simulink library "LIB_DYN"  (Simulink 8.8)
settings: Solver=ode45  StartTime=0.0  StopTime=10.0  RelTol=1e-3  EnableMultiTasking=on
libraries: LIB_ROT x5
settings Model: Creator=alger  LastModifiedBy=alger

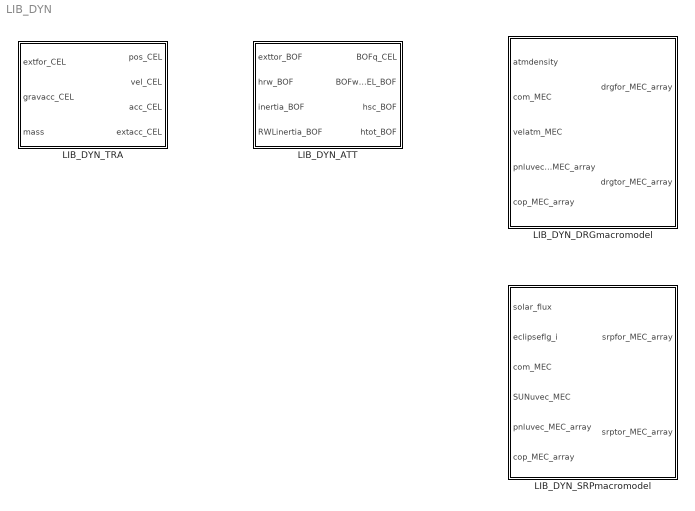
== system LIB_DYN ==
  LIB_DYN_ATT : Subsystem  mask(Integrates Attitude States){BOFq_CEL_ini=0, h_BOF_ini=0, zero_tol=0}
      mask prompts: BOFq_CEL_ini "inital Body to Cel Frame Quaternion"; h_BOF_ini "inital angular momentum of body frame"; zero_tol "near zero tolerance"
      mask help:
      | Integrates attitude states of a spacecraft (or part of a spacecraft) in the Body Frame w.r.t an inertial celestial frame
      |
      | Inputs
      | exttor_BOF: exteral torques acting on the spacecraft [N]
      | hrw_BOF: momentum exchange with other components of the spacecraft e.g. reaction wheels [Nms]
      | inertia_BOF: current inertia of the spacecraft in body frame[kg/m^2]
      | RWinertia_BOF: current inertia of other components of the spacecraft e.g. reaction wheels[kg/m^2]
      |
      | Outputs
      | BOFq_CEL: quaterion relating celestial and body frames[-]
      | BOFw_rel_CEL_BOF: rates of rotation between celestial and body frames expressed in terms of the BOF frame [rad/s]
      | hsc_BOF: angular momentum of spaceccraft (e.g. no momentum from reaction wheels)[Nms]
      | htot_BOF:angular momentum of spacecraft and any exchanged momentum[Nms]
  "LIB_DYN_DRGmacromodel " : Subsystem  mask{N=6, pnlarea_array=[0.1, 0.1, 0.1, 0.1, 0.1, 0.1], pnlcd_array=[0.5, 0.5, 0.5, 0.5, 0.5, 0.5]}
      mask prompts: N "Number of panels"; pnlarea_array "Surface area for each panel"; pnlcd_array "Drag coeffiecent for each panel"
  LIB_DYN_SRPmacromodel : Subsystem  mask{N=6, C=0, pnlarea_array=[0.1, 0.1, 0.1, 0.1, 0.1, 0.1], pnlcrd_array=[0.15, 0.15, 0.15, 0.15, 0.15, 0.15], pnlcrs_array=[0.75, 0.75, 0.75, 0.75, 0.75, 0.75]}
      mask prompts: N "Number of panels"; C "Speed of light constant (m/s)"; pnlarea_array "Surface area for each panel"; pnlcrd_array "diffuse coefficentfor each panel"; pnlcrs_array "specular coefficent for each panel"
      mask help: absorbed coefficent is computed based on 1-(crd +crs)
  LIB_DYN_TRA : Subsystem  mask(Integrates translational states){pos_CEL_ini=0, vel_CEL_ini=0}
      mask prompts: pos_CEL_ini "Initial position in inertial celestial frame  [m]"; vel_CEL_ini "Intial velocity in an inertial celestial frame[m/s]"
      mask help:
      | integrates translational states in an inertial celestial frame using integrator blocks from matlab.
      |
      | Inputs
      | extfor_CEL: External forces acting on the spacecraft expressed in a inertial Celestial frame [N]
      | gravacc_CEL: Acceleration due to gravity of the planetary body the spacecraft is orbiting [m/s^2]
      | mass:  mass of the spacecraft
      |
      | Ouptuts
      | pos_CEL: integrated position of spacecraft in an inertial celestial frame [m]
      | vel_CEL: integrated velocity of spacecraft in an inertial celestial frame[m/s]
      | acc_CEL: net acceleration of spacecraft in an inertial celestial frame[m/^s]
      | extacc_CEL: accleration of spacecraft due to external forces only in an inertial celestial frame[m/s^2]

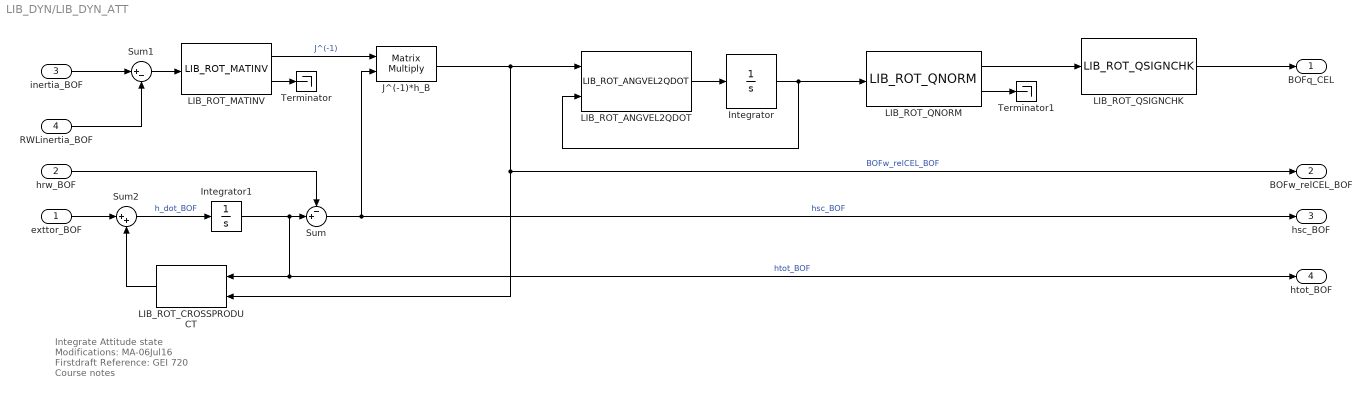
== system LIB_DYN/LIB_DYN_ATT ==
  note: Integrate Attitude state
      |
      | Modifications:
      | MA-06Jul16 Firstdraft
      |
      | Reference:
      | GEI 720 Course notes
  exttor_BOF : Inport  PortDimensions=3
  hrw_BOF : Inport  Port=2  PortDimensions=3
  inertia_BOF : Inport  Port=3  PortDimensions=[3,3]
  RWLinertia_BOF : Inport  Port=4  PortDimensions=[3,3]
  Integrator : Integrator  InitialCondition=BOFq_CEL_ini
  Integrator1 : Integrator  InitialCondition=h_BOF_ini
  J^(-1)*h_B : Product  Multiplication=Matrix(*)  RndMeth=Zero
  LIB_ROT_ANGVEL2QDOT : LIB_ROT/LIB_ROT_ANGVEL2QDOT
  LIB_ROT_CROSSPRODUCT : LIB_ROT/LIB_ROT_CROSSPRODUCT
  "LIB_ROT_MATINV " : LIB_ROT/LIB_ROT_MATINV   tol=zero_tol
  LIB_ROT_QNORM : LIB_ROT/LIB_ROT_QNORM  zero_tol=zero_tol
  LIB_ROT_QSIGNCHK : LIB_ROT/LIB_ROT_QSIGNCHK  tol=zero_tol
  Sum : Sum  Inputs=-+|
  Sum1 : Sum  Inputs=|+-
  Sum2 : Sum  Inputs=|++
  Terminator : Terminator
  Terminator1 : Terminator
  BOFq_CEL : Outport  PortDimensions=4
  BOFw_relCEL_BOF : Outport  Port=2  PortDimensions=3
  hsc_BOF : Outport  Port=3  PortDimensions=3
  htot_BOF : Outport  Port=4  PortDimensions=3
  wires:
  inertia_BOF/1 -> Sum1/1
  RWLinertia_BOF/1 -> Sum1/2
  "LIB_ROT_MATINV "/1 -> J^(-1)*h_B/1  "J^(-1)"
  Sum1/1 -> "LIB_ROT_MATINV "/1
  hrw_BOF/1 -> Sum/1
  exttor_BOF/1 -> Sum2/1
  Sum2/1 -> Integrator1/1  "h_dot_BOF"
  Integrator1/1 -> LIB_ROT_CROSSPRODUCT/1, htot_BOF/1, Sum/2  "htot_BOF"
  J^(-1)*h_B/1 -> BOFw_relCEL_BOF/1, LIB_ROT_CROSSPRODUCT/2, LIB_ROT_ANGVEL2QDOT/1  "BOFw_relCEL_BOF"
  Sum/1 -> J^(-1)*h_B/2, hsc_BOF/1  "hsc_BOF"
  LIB_ROT_CROSSPRODUCT/1 -> Sum2/2
  "LIB_ROT_MATINV "/2 -> Terminator/1
  LIB_ROT_ANGVEL2QDOT/1 -> Integrator/1
  Integrator/1 -> LIB_ROT_QNORM/1, LIB_ROT_ANGVEL2QDOT/2
  LIB_ROT_QNORM/1 -> LIB_ROT_QSIGNCHK/1
  LIB_ROT_QNORM/2 -> Terminator1/1
  LIB_ROT_QSIGNCHK/1 -> BOFq_CEL/1

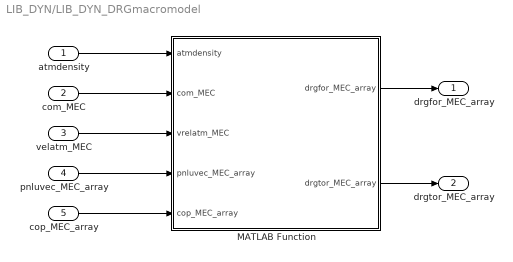
== system LIB_DYN/LIB_DYN_DRGmacromodel  ==
  atmdensity : Inport  Unit=kg/m^3  PortDimensions=1
  com_MEC : Inport  Port=2  Unit=m  PortDimensions=3
  velatm_MEC : Inport  Port=3  PortDimensions=3
  pnluvec_MEC_array : Inport  Port=4  PortDimensions=[3, N]  LockScale=on
  cop_MEC_array : Inport  Port=5  Unit=m  PortDimensions=[3, N]
  MATLAB Function : MATLAB Function  TreatAsAtomicUnit=on
  drgfor_MEC_array : Outport  PortDimensions=[3, N]
  drgtor_MEC_array : Outport  Port=2  PortDimensions=[3, N]
  wires:
  cop_MEC_array/1 -> MATLAB Function/5(cop_MEC_array)
  atmdensity/1 -> MATLAB Function/1(atmdensity)
  com_MEC/1 -> MATLAB Function/2(com_MEC)
  velatm_MEC/1 -> MATLAB Function/3(vrelatm_MEC)
  pnluvec_MEC_array/1 -> MATLAB Function/4(pnluvec_MEC_array)
  MATLAB Function/2(drgtor_MEC_array) -> drgtor_MEC_array/1
  MATLAB Function/1(drgfor_MEC_array) -> drgfor_MEC_array/1

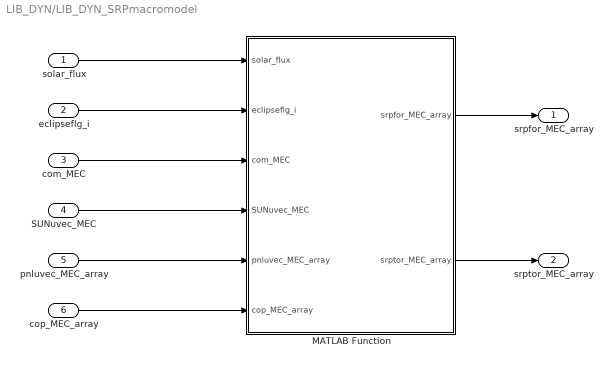
== system LIB_DYN/LIB_DYN_SRPmacromodel ==
  solar_flux : Inport  Unit=kg/m^3  PortDimensions=1
  eclipseflg_i : Inport  Port=2  Unit=kg/m^3  PortDimensions=1
  com_MEC : Inport  Port=3  Unit=m  PortDimensions=3
  SUNuvec_MEC : Inport  Port=4  PortDimensions=3
  pnluvec_MEC_array : Inport  Port=5  PortDimensions=[3, N]  LockScale=on
  cop_MEC_array : Inport  Port=6  Unit=m  PortDimensions=[3, N]
  MATLAB Function : MATLAB Function  TreatAsAtomicUnit=on
  srpfor_MEC_array : Outport  PortDimensions=[3, N]
  srptor_MEC_array : Outport  Port=2  PortDimensions=[3, N]
  wires:
  MATLAB Function/1(srpfor_MEC_array) -> srpfor_MEC_array/1
  MATLAB Function/2(srptor_MEC_array) -> srptor_MEC_array/1
  pnluvec_MEC_array/1 -> MATLAB Function/5(pnluvec_MEC_array)
  SUNuvec_MEC/1 -> MATLAB Function/4(SUNuvec_MEC)
  com_MEC/1 -> MATLAB Function/3(com_MEC)
  solar_flux/1 -> MATLAB Function/1(solar_flux)
  cop_MEC_array/1 -> MATLAB Function/6(cop_MEC_array)
  eclipseflg_i/1 -> MATLAB Function/2(eclipseflg_i)

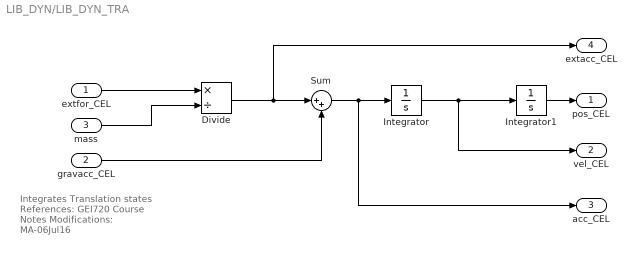
== system LIB_DYN/LIB_DYN_TRA ==
  note: Integrates Translation states
      |
      |
      | References:
      | GEI720 Course Notes
      |
      | Modifications:
      | MA-06Jul16
  extfor_CEL : Inport  PortDimensions=3
  gravacc_CEL : Inport  Port=2  PortDimensions=3
  mass : Inport  Port=3  PortDimensions=1
  Divide : Product  Inputs=*/
  Integrator : Integrator  InitialCondition=vel_CEL_ini
  Integrator1 : Integrator  InitialCondition=pos_CEL_ini
  Sum : Sum  Inputs=|++
  pos_CEL : Outport
  vel_CEL : Outport  Port=2  PortDimensions=3
  acc_CEL : Outport  Port=3  PortDimensions=3
  extacc_CEL : Outport  Port=4  PortDimensions=3
  wires:
  extfor_CEL/1 -> Divide/1
  gravacc_CEL/1 -> Sum/2
  Integrator/1 -> vel_CEL/1, Integrator1/1
  Integrator1/1 -> pos_CEL/1
  mass/1 -> Divide/2
  Divide/1 -> Sum/1, extacc_CEL/1
  Sum/1 -> acc_CEL/1, Integrator/1

== matlab function LIB_DYN_SRPmacromodel/MATLAB Function ==
  data: solar_flux input double; eclipseflg_i input double; com_MEC input double; SUNuvec_MEC input double; srpfor_MEC_array output double size=[3,N]; pnluvec_MEC_array input double; cop_MEC_array input double; N parameter double; C parameter double; srptor_MEC_array output double size=[3,N]; pnlarea_array parameter double; pnlcrd_array parameter double; pnlcrs_array parameter double
function [srpfor_MEC_array, srptor_MEC_array]  = LIB_DYN_SRPmacroplate( ...
                                                  solar_flux,         ...
                                                  eclipseflg_i,       ...
                                                  com_MEC,            ...
                                                  SUNuvec_MEC,        ...
                                                  pnluvec_MEC_array,  ...
                                                  cop_MEC_array,      ...
                                                  N,                  ...  
                                                  C,              ...  
                                                  pnlarea_array,      ...
                                                  pnlcrd_array,       ...
                                                  pnlcrs_array)       ...
  %#codegen
  srpfor_MEC_array = zeros(3,N);
  srptor_MEC_array = zeros(3,N);
  for i = 1:N
    srpfor_MEC_array(:,i) = dynsrpfor_pnl(solar_flux,           ...
                                          SUNuvec_MEC,          ...
                                          pnluvec_MEC_array(:,i), ...
                                          eclipseflg_i,         ...
                                          C,                    ...
                                          pnlarea_array(i),     ...
                                          pnlcrd_array(i),      ...
                                          pnlcrs_array(i));

                                  
    srptor_MEC_array(:,i) = dynfor2tor_pnl( srpfor_MEC_array(:,i),  ...
                                            com_MEC,                ...
                                            cop_MEC_array(:,i));                                                  
  end
end

== matlab function LIB_DYN_DRGmacromodel /MATLAB Function ==
  data: atmdensity input double; drgfor_MEC_array output double size=[3,N]; com_MEC input double; vrelatm_MEC input double; pnluvec_MEC_array input double; cop_MEC_array input double; drgtor_MEC_array output double size=[3,N]; pnlcd_array parameter double; pnlarea_array parameter double; N parameter double
function [drgfor_MEC_array, drgtor_MEC_array]  = LIB_DYN_DRGmacroplate( ...
                                                  atmdensity,           ...
                                                  com_MEC,              ...
                                                  vrelatm_MEC,          ...
                                                  pnluvec_MEC_array,    ...
                                                  cop_MEC_array,        ...
                                                  pnlcd_array,          ...
                                                  pnlarea_array,        ...
                                                  N)

  %#codegen
  drgfor_MEC_array = zeros(3,N);
  drgtor_MEC_array = zeros(3,N);
  for i = 1:N
    drgfor_MEC_array(:,i) = dyndrgfor_pnl(                  ...
                                    atmdensity,             ...
                                    vrelatm_MEC,            ...
                                    pnluvec_MEC_array(:,i), ...
                                    pnlarea_array(i),       ...
                                    pnlcd_array(i));
                                  
    drgtor_MEC_array(:,i) = dynfor2tor_pnl(                 ...
                                    drgfor_MEC_array(:,i),  ...
                                    com_MEC,                ...
                                    cop_MEC_array(:,i));                                                  
  end
end
